simulink model "prob4_week2"  (R2020b)
settings: Solver=VariableStepAuto  StartTime=0.0  StopTime=10.0  RelTol=1e-3
undefined symbols (not defined in the file): b, J, ke, kt, L, R
settings Model: Creator=Pulkit Khandelwal  LastModifiedBy=Pulkit Khandelwal

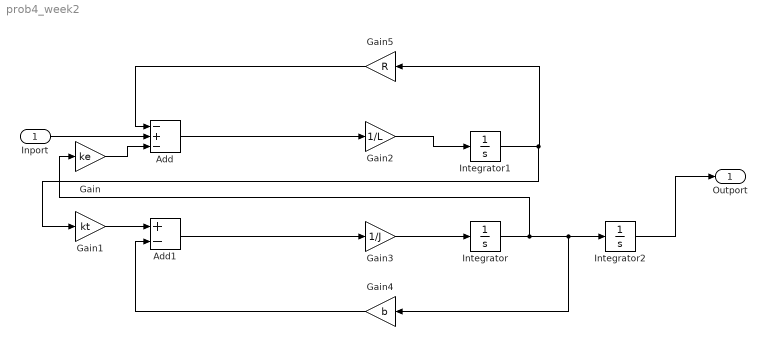
== system prob4_week2 ==
  Inport : Inport
  Add : Sum  Inputs=-+-
  Add1 : Sum  Inputs=+-
  Gain : Gain  Gain=ke
  Gain1 : Gain  Gain=kt
  Gain2 : Gain  Gain=1/L
  Gain3 : Gain  Gain=1/J
  Gain4 : Gain  Gain=b
  Gain5 : Gain  Gain=R
  Integrator : Integrator
  Integrator1 : Integrator
  Integrator2 : Integrator
  Outport : Outport
  wires:
  Gain2/1 -> Integrator1/1
  Inport/1 -> Add/2
  Integrator2/1 -> Outport/1
  Gain1/1 -> Add1/1
  Add/1 -> Gain2/1
  Gain4/1 -> Add1/2
  Gain/1 -> Add/3
  Integrator1/1 -> Gain5/1, Gain1/1
  Integrator/1 -> Integrator2/1, Gain4/1, Gain/1
  Add1/1 -> Gain3/1
  Gain5/1 -> Add/1
  Gain3/1 -> Integrator/1
